simulink model "compare_different_quaternion_integration"  (R2024a)
settings: Solver=FixedStepAuto  StartTime=0.0  StopTime=10.0  FixedStep=0.01  RelTol=1e-3
undefined symbols (not defined in the file or in its folder): e0_0, e1_0, e2_0, e3_0
libraries: sharedtransform x2, sharedutil x1, shared6dofsys x1
settings Model: Creator=bemran  LastModifiedBy=bemran

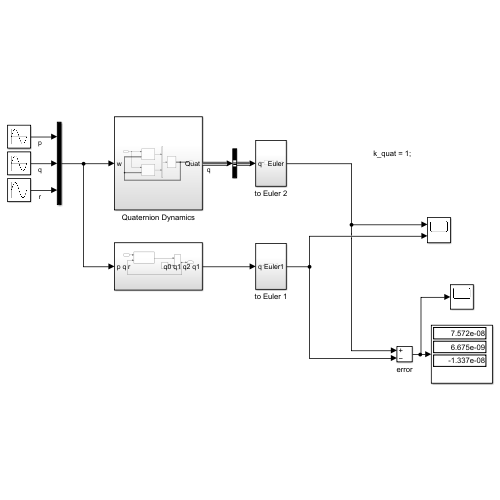
[thumbnail: Simulink's stored preview of the top-level diagram]
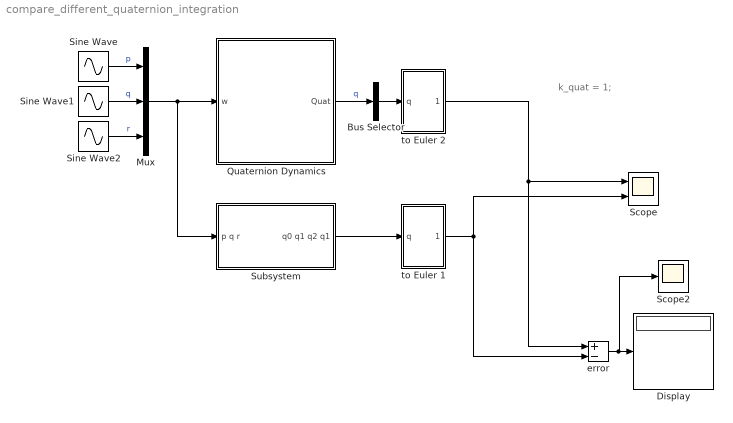
== system compare_different_quaternion_integration ==
  note: k_quat = 1;
  Bus Selector : BusSelector  OutputSignals=q0,q_vec.q1,q_vec.q2,q_vec.q3  OutputAsBus=on
  Display : Display
  Mux : Mux  Inputs=3
  Quaternion Dynamics : Subsystem
  Scope : Scope  NumInputPorts=2
  Scope2 : Scope
  Sine Wave : Sin  SampleTime=0
  Sine Wave1 : Sin  Amplitude=2  Frequency=5  Phase=-1  SampleTime=0
  Sine Wave2 : Sin  Amplitude=-1  Frequency=10  Phase=1  SampleTime=0
  Subsystem : Subsystem
  error : Sum  Inputs=+-
  to Euler 1 : Subsystem
  to Euler 2 : Subsystem
  wires:
  Subsystem/1(q0 q1 q2 q1) -> to Euler 1/1(q)
  Quaternion Dynamics/1(Quat) -> Bus Selector/1  "q"
  Sine Wave/1 -> Mux/1  "p"
  Sine Wave1/1 -> Mux/2  "q"
  Sine Wave2/1 -> Mux/3  "r"
  Mux/1 -> Subsystem/1(p q r), Quaternion Dynamics/1(w)
  Bus Selector/1 -> to Euler 2/1(q)
  to Euler 1/1(Euler1) -> error/2, Scope/2
  to Euler 2/1(Euler) -> error/1, Scope/1
  error/1 -> Scope2/1, Display/1

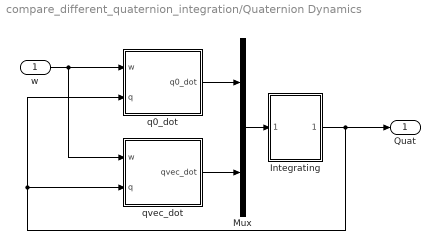
== system compare_different_quaternion_integration/Quaternion Dynamics ==
  w : Inport
  Integrating : Subsystem
  Mux : Mux  Inputs=2
  q0_dot : Subsystem
  qvec_dot : Subsystem
  Quat : Outport  OutDataTypeStr=double  VectorParamsAs1DForOutWhenUnconnected=off
  wires:
  Integrating/1(Quat) -> Quat/1, q0_dot/2(q), qvec_dot/2(q)
  qvec_dot/1(qvec_dot) -> Mux/2
  q0_dot/1(q0_dot) -> Mux/1
  w/1 -> qvec_dot/1(w), q0_dot/1(w)
  Mux/1 -> Integrating/1(qdot)

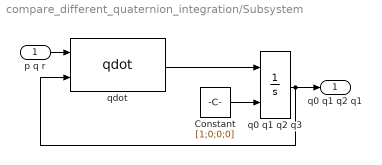
== system compare_different_quaternion_integration/Subsystem ==
  p q r : Inport
  Constant : Constant  Value=[1;0;0;0]
  q0 q1 q2 q3 : Integrator  InitialConditionSource=external  InitialCondition=[e0_0 e1_0 e2_0 e3_0]
  qdot : shared6dofsys/DCM & Euler Angles (Quaternion)/qdot  SystemSampleTime=-1  VariantActivationTime=update diagram  AllowFlexibleInterface=on  Latency=0  AutoFrameSizeCalculation=off
  q0 q1 q2 q1 : Outport
  wires:
  qdot/1 -> q0 q1 q2 q3/1
  Constant/1 -> q0 q1 q2 q3/2
  p q r/1 -> qdot/1
  q0 q1 q2 q3/1 -> qdot/2, q0 q1 q2 q1/1

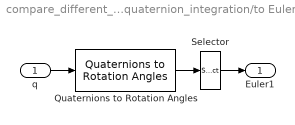
== system compare_different_quaternion_integration/to Euler 1 ==
  q : Inport
  Quaternions to Rotation Angles : sharedtransform/Quaternions to Rotation Angles  rotationOrder=ZYX  aMode=aMode
  Selector : Selector  InputPortWidth=3  IndexOptions=Index vector (dialog)  Indices=[3 2 1]  OutputSizes=1
  Euler1 : Outport  OutDataTypeStr=double  VectorParamsAs1DForOutWhenUnconnected=off
  wires:
  Quaternions to Rotation Angles/1 -> Selector/1
  Selector/1 -> Euler1/1
  q/1 -> Quaternions to Rotation Angles/1

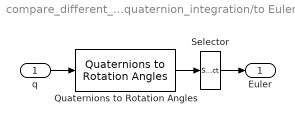
== system compare_different_quaternion_integration/to Euler 2 ==
  q : Inport
  Quaternions to Rotation Angles : sharedtransform/Quaternions to Rotation Angles  rotationOrder=ZYX  aMode=aMode
  Selector : Selector  InputPortWidth=3  IndexOptions=Index vector (dialog)  Indices=[3 2 1]  OutputSizes=1
  Euler : Outport  OutDataTypeStr=double  VectorParamsAs1DForOutWhenUnconnected=off
  wires:
  Quaternions to Rotation Angles/1 -> Selector/1
  Selector/1 -> Euler/1
  q/1 -> Quaternions to Rotation Angles/1

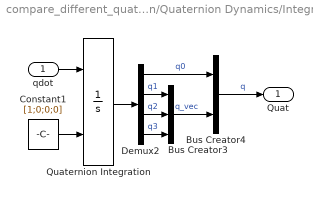
== system compare_different_quaternion_integration/Quaternion Dynamics/Integrating ==
  qdot : Inport
  Bus Creator3 : BusCreator  Inputs=3
  Bus Creator4 : BusCreator  Inputs=2
  Constant1 : Constant  Value=[1;0;0;0]
  Demux2 : Demux
  Quaternion Integration : Integrator  InitialConditionSource=external  InitialCondition=[e0_0 e1_0 e2_0 e3_0]
  Quat : Outport  OutDataTypeStr=double  VectorParamsAs1DForOutWhenUnconnected=off
  wires:
  Bus Creator3/1 -> Bus Creator4/2  "q_vec"
  Bus Creator4/1 -> Quat/1  "q"
  Demux2/3 -> Bus Creator3/2  "q2"
  Quaternion Integration/1 -> Demux2/1
  Demux2/1 -> Bus Creator4/1  "q0"
  Demux2/2 -> Bus Creator3/1  "q1"
  qdot/1 -> Quaternion Integration/1
  Demux2/4 -> Bus Creator3/3  "q3"
  Constant1/1 -> Quaternion Integration/2

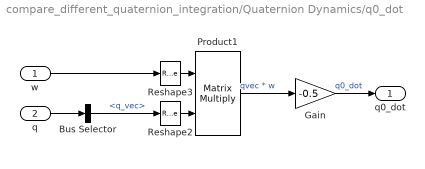
== system compare_different_quaternion_integration/Quaternion Dynamics/q0_dot ==
  w : Inport  OutDataTypeStr=double
  q : Inport  Port=2
  Bus Selector : BusSelector  OutputSignals=q_vec
  Gain : Gain  Gain=-0.5
  Product1 : Product  Inputs=**  Multiplication=Matrix(*)  SaturateOnIntegerOverflow=on  OutDataTypeStr=Inherit: Same as first input
  Reshape2 : Reshape  OutputDimensionality=Column vector (2-D)
  Reshape3 : Reshape  OutputDimensionality=Row vector (2-D)
  q0_dot : Outport
  wires:
  Bus Selector/1 -> Reshape2/1  "<q_vec>"
  Reshape2/1 -> Product1/2
  w/1 -> Reshape3/1
  Reshape3/1 -> Product1/1
  Gain/1 -> q0_dot/1  "q0_dot"
  Product1/1 -> Gain/1  "qvec * w"
  q/1 -> Bus Selector/1

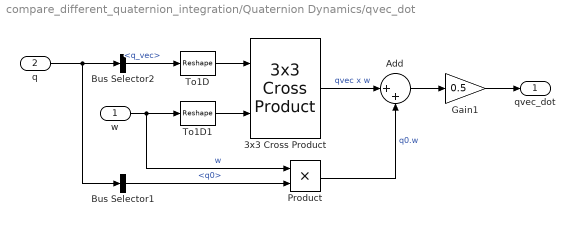
== system compare_different_quaternion_integration/Quaternion Dynamics/qvec_dot ==
  w : Inport  OutDataTypeStr=double
  q : Inport  Port=2
  3x3 Cross Product : sharedutil/3x3 Cross Product  aMode=aMode
  Add : Sum  Inputs=|++
  Bus Selector1 : BusSelector  OutputSignals=q0
  Bus Selector2 : BusSelector  OutputSignals=q_vec
  Gain1 : Gain  Gain=0.5
  Product : Product
  To1D : Reshape
  To1D1 : Reshape
  qvec_dot : Outport
  wires:
  w/1 -> Product/1, To1D1/1  "w"
  Add/1 -> Gain1/1
  Bus Selector1/1 -> Product/2  "<q0>"
  To1D1/1 -> 3x3 Cross Product/2
  q/1 -> Bus Selector1/1, Bus Selector2/1
  To1D/1 -> 3x3 Cross Product/1
  Bus Selector2/1 -> To1D/1  "<q_vec>"
  3x3 Cross Product/1 -> Add/1  "qvec x w"
  Product/1 -> Add/2  "q0.w"
  Gain1/1 -> qvec_dot/1
